simulink model "Encoder_Sim3"  (R2024b)
settings: Solver=FixedStepAuto  StartTime=0.0  StopTime=inf  FixedStep=0.01  RelTol=1e-3  EnableMultiTasking=on
libraries: stm32g4xxblockslib x4, stm32f4xxblockslib x3
settings Model: STM32="{\"EncoderBlockForG4\":[{\"ID\":\"Encoder_Sim3:80\"},{\"ID\":\"Encoder_Sim3:125\"},{\"ID\":\"Encoder_Sim3:137\"},{\"ID\":\"Encoder_Sim3:146\"}],\"DigitalPortRead\":[{\"ID\":\"Encoder_Sim3:75\"},{\"ID\":\"Encoder_Sim3:123\"},{\"ID\":\"Encoder_Sim3:135\"}]}"  SimulationMode=external  Creator=chant  LastModifiedBy=chant
settings OptimizationCC: DefaultParameterBehavior=Inlined  EnhancedBackFolding=on  PassReuseOutputArgsAs=Individual arguments  ZeroExternalMemoryAtStartup=off  ZeroInternalMemoryAtStartup=off  MaxStackSize=512  OptimizeBlockOrder=speed  DifferentSizesBufferReuse=on  OptimizationCustomize=off  EfficientTunableParamExpr=on
settings DebuggingCC: ParameterTunabilityLossMsg=error
settings HardwareCC: ProdBitPerPointer=32  ProdBitPerSizeT=32  ProdBitPerPtrDiffT=32  ProdLargestAtomicInteger=Long  ProdLargestAtomicFloat=Double  ProdWordSize=32  ProdLongLongMode=on  ProdHWDeviceType=ARM Compatible->ARM Cortex-M
settings SFSimCC: MATLABDynamicMemAlloc=off
settings RTWCC: Description=Embedded Coder  SystemTargetFile=ert.tlc  HardwareBoard=STM32G4xx Based  TemplateMakefile=ert_default_tmf  Toolchain=GNU Tools for ARM Embedded Processors
settings CodeAppCC: ForceParamTrailComments=on  IgnoreCustomStorageClasses=off  OperatorAnnotations=on  SimulinkDataObjDesc=on  SFDataObjDesc=on  InsertBlockDesc=on
settings ERTTargetCC: TargetLangStandard=C99 (ISO)  CodeReplacementLibrary=ARM Cortex-M  ExtModeTransport=3  ExtModeStaticAlloc=on  ExtModeStaticAllocSize=2048  ExtModeMexFile=ext_xcp  ExtModeIntrfLevel=Level2 - Open

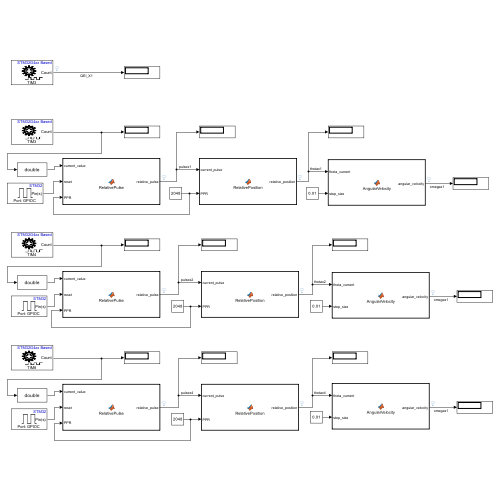
[thumbnail: Simulink's stored preview of the top-level diagram]
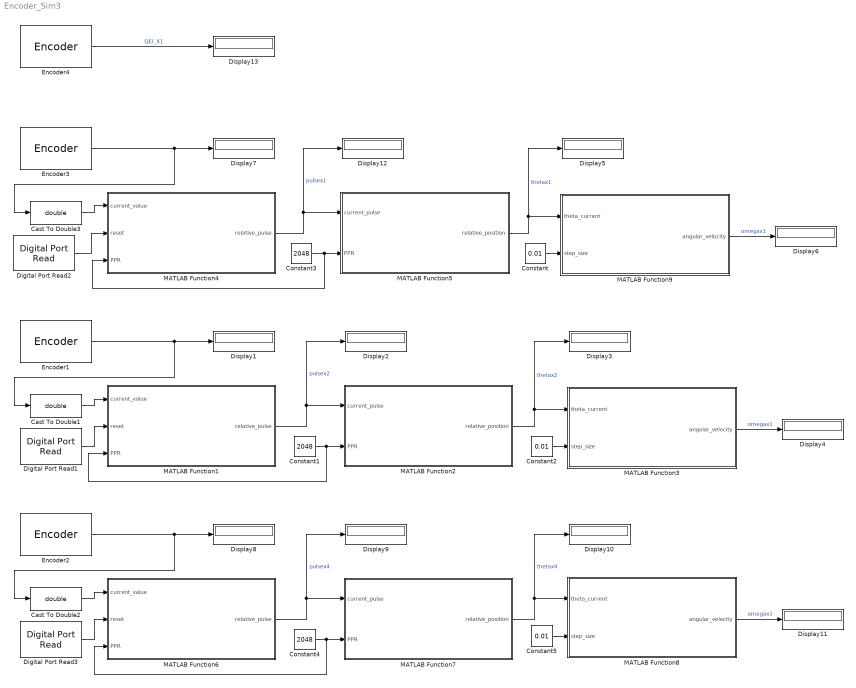
== system Encoder_Sim3 ==
  Cast To Double1 : DataTypeConversion  OutDataTypeStr=double  SaturateOnIntegerOverflow=off  RndMeth=Floor
  Cast To Double2 : DataTypeConversion  OutDataTypeStr=double  SaturateOnIntegerOverflow=off  RndMeth=Floor
  Cast To Double3 : DataTypeConversion  OutDataTypeStr=double  SaturateOnIntegerOverflow=off  RndMeth=Floor
  Constant : Constant  Value=0.01
  Constant1 : Constant  Value=2048
  Constant2 : Constant  Value=0.01
  Constant3 : Constant  Value=2048
  Constant4 : Constant  Value=2048
  Constant5 : Constant  Value=0.01
  Digital Port Read1 : stm32f4xxblockslib/Digital Port Read  PortName=GPIOC  PinNumber=[13]  ReadOperation=on  IOAsArray=on  SampleTime=-1  EnableSimPort=off  hoistedMaskSrc=ECSoC/ECSimCodegen/Digital Port Read
      settings: LibrarySourceBlock=stm32g4xxblockslib/Digital Port Read
  Digital Port Read2 : stm32f4xxblockslib/Digital Port Read  PortName=GPIOC  PinNumber=[13]  ReadOperation=on  IOAsArray=on  SampleTime=-1  EnableSimPort=off  hoistedMaskSrc=ECSoC/ECSimCodegen/Digital Port Read
      settings: LibrarySourceBlock=stm32g4xxblockslib/Digital Port Read
  Digital Port Read3 : stm32f4xxblockslib/Digital Port Read  PortName=GPIOC  PinNumber=[13]  ReadOperation=on  IOAsArray=on  SampleTime=-1  EnableSimPort=off  hoistedMaskSrc=ECSoC/ECSimCodegen/Digital Port Read
      settings: LibrarySourceBlock=stm32g4xxblockslib/Digital Port Read
  Display{1..13} (13 alike) : Display
  Encoder1 : stm32g4xxblockslib/Encoder  TimerModule=TIM4  EnableResetInput=off  OutputCountAfterFirstIndex=off  OutputValidIndex=off  OutputDirection=off  OutputStatus=off  SampleTime=-1
  Encoder2 : stm32g4xxblockslib/Encoder  TimerModule=TIM8  EnableResetInput=off  OutputCountAfterFirstIndex=off  OutputValidIndex=off  OutputDirection=off  OutputStatus=off  SampleTime=-1
  Encoder3 : stm32g4xxblockslib/Encoder  TimerModule=TIM3  EnableResetInput=off  OutputCountAfterFirstIndex=off  OutputValidIndex=off  OutputDirection=off  OutputStatus=off  SampleTime=-1
  Encoder4 : stm32g4xxblockslib/Encoder  TimerModule=TIM3  EnableResetInput=off  OutputCountAfterFirstIndex=off  OutputValidIndex=off  OutputDirection=off  OutputStatus=off  SampleTime=-1
  MATLAB Function1 : MATLAB Function  TreatAsAtomicUnit=on
  MATLAB Function2 : MATLAB Function  TreatAsAtomicUnit=on
  MATLAB Function3 : MATLAB Function  TreatAsAtomicUnit=on
  MATLAB Function4 : MATLAB Function  TreatAsAtomicUnit=on
  MATLAB Function5 : MATLAB Function  TreatAsAtomicUnit=on
  MATLAB Function6 : MATLAB Function  TreatAsAtomicUnit=on
  MATLAB Function7 : MATLAB Function  TreatAsAtomicUnit=on
  MATLAB Function8 : MATLAB Function  TreatAsAtomicUnit=on
  MATLAB Function9 : MATLAB Function  TreatAsAtomicUnit=on
  wires:
  Cast To Double3/1 -> MATLAB Function4/1(current_value)
  MATLAB Function9/1(angular_velocity) -> Display6/1  "omegax1"
  MATLAB Function5/1(relative_position) -> Display5/1, MATLAB Function9/1(theta_current)  "thetax1"
  Digital Port Read2/1 -> MATLAB Function4/2(reset)
  Encoder3/1 -> Display7/1, Cast To Double3/1
  Constant3/1 -> MATLAB Function4/3(PPR), MATLAB Function5/2(PPR)
  MATLAB Function4/1(relative_pulse) -> MATLAB Function5/1(current_pulse), Display12/1  "pulsex1"
  Constant/1 -> MATLAB Function9/2(step_size)
  Encoder1/1 -> Cast To Double1/1, Display1/1
  Digital Port Read1/1 -> MATLAB Function1/2(reset)
  Cast To Double1/1 -> MATLAB Function1/1(current_value)
  MATLAB Function1/1(relative_pulse) -> Display2/1, MATLAB Function2/1(current_pulse)  "pulsex2"
  Constant1/1 -> MATLAB Function1/3(PPR), MATLAB Function2/2(PPR)
  Constant2/1 -> MATLAB Function3/2(step_size)
  MATLAB Function2/1(relative_position) -> MATLAB Function3/1(theta_current), Display3/1  "thetax2"
  MATLAB Function3/1(angular_velocity) -> Display4/1  "omegax1"
  Cast To Double2/1 -> MATLAB Function6/1(current_value)
  Digital Port Read3/1 -> MATLAB Function6/2(reset)
  Encoder2/1 -> Display8/1, Cast To Double2/1
  Constant4/1 -> MATLAB Function6/3(PPR), MATLAB Function7/2(PPR)
  MATLAB Function6/1(relative_pulse) -> MATLAB Function7/1(current_pulse), Display9/1  "pulsex4"
  MATLAB Function8/1(angular_velocity) -> Display11/1  "omegax1"
  MATLAB Function7/1(relative_position) -> Display10/1, MATLAB Function8/1(theta_current)  "thetax4"
  Constant5/1 -> MATLAB Function8/2(step_size)
  Encoder4/1 -> Display13/1  "QEI_X1"

== matlab function Encoder_Sim3/MATLAB Function1 ==
  data: current_value input; relative_pulse output; reset input; PPR input
function relative_pulse = RelativePulse(current_value, reset, PPR)
    % Persistent variables to retain values across function calls
    persistent prev_value rollover_count max_value reset_flag pulse_offset

    % Initialize persistent variables on the first function call
    if isempty(prev_value)
        prev_value = 0;
    end
    if isempty(rollover_count)
        rollover_count = 0;
    end
    if isempty(max_value)
        max_value = 65535-(mod(65535, PPR)); % Set a default max value if not provided
    end
    if isempty(reset_flag)
        reset_flag = 0; % Track if reset has been triggered
    end
    if isempty(pulse_offset)
        pulse_offset = 0; % Offset to correct pulse on reset
    end

    % Set a default value for relative_pulse to avoid "undefined" errors
    relative_pulse = 0;

    % Threshold to detect overflow/underflow
    threshold = max_value / 2;

    % Detect overflow (encoder wrapped from high to low)
    if current_value < prev_value && (prev_value - current_value) > threshold
        rollover_count = rollover_count + 1;

    % Detect underflow (encoder wrapped from low to high)
    elseif current_value > prev_value && (current_value - prev_value) > threshold
        rollover_count = rollover_count - 1;
    end

    % Calculate true count (absolute pulse count)
    true_count = rollover_count * (max_value + 1) + current_value;

    % Homing logic: align to zero on reset
    if reset == 1 && reset_flag == 0
        % Set pulse_offset to the current true_count, so relative_pulse resets to 0
        pulse_offset = true_count;
        reset_flag = 1;  % Set the reset flag to avoid multiple resets
    elseif reset == 0
        % Clear the reset flag once the button is released
        reset_flag = 0;
    end

    % Calculate relative pulse with offset compensation
    relative_pulse = true_count - pulse_offset;

    % Update previous value for the next call
    prev_value = current_value;
end

== matlab function Encoder_Sim3/MATLAB Function2 ==
  data: current_pulse input; relative_position output; PPR input
function relative_position = RelativePosition(current_pulse, PPR)
    % Persistent variables to retain values across function calls
    persistent prev_pulse rollover_count max_value

    % Initialize persistent variables on the first function call
    if isempty(prev_pulse)
        prev_pulse = 0;
    end
    if isempty(rollover_count)
        rollover_count = 0;
    end
    if isempty(max_value)
        max_value = 23; % Maximum value for a 16-bit encoder
    end

    % Detect overflow (encoder wrapped from max to 0)
    if current_pulse < prev_pulse && (prev_pulse - current_pulse) > (max_value / 2)
        rollover_count = rollover_count + 1;

    % Detect underflow (encoder wrapped from 0 to max)
    elseif current_pulse > prev_pulse && (current_pulse - prev_pulse) > (max_value / 2)
        rollover_count = rollover_count - 1;
    end

    % Calculate true count (relative pulse)
    true_count = rollover_count * (max_value + 1) + current_pulse;

    % Calculate the relative position in radians (unlimited)
    relative_position = true_count * (2 * pi / PPR); % Convert to radians

    % Update previous value for the next call
    prev_pulse = current_pulse;
end

== matlab function Encoder_Sim3/MATLAB Function3 ==
  data: theta_current input; angular_velocity output; step_size input
function angular_velocity = AngularVelocity(theta_current, step_size)
    % Calculate angular velocity based on the fixed step size
    % Inputs:
    %   theta_current: The current angular position (in degrees)
    %   step_size: The fixed time step size (in seconds)

    % Persistent variable to store the previous position
    persistent theta_previous;

    % Initialize on the first call
    if isempty(theta_previous)
        theta_previous = theta_current;
        angular_velocity = 0;  % Start with zero angular velocity
        return;  % Exit on the first call
    end

    % Calculate the change in position (delta_theta)
    delta_theta = theta_current - theta_previous;

    % Calculate angular velocity (degrees per second)
    angular_velocity = delta_theta / step_size;

    % Update the previous position for the next call
    theta_previous = theta_current;
end

== matlab function Encoder_Sim3/MATLAB Function4 ==
  data: current_value input; relative_pulse output; reset input; PPR input
function relative_pulse = RelativePulse(current_value, reset, PPR)
    % Persistent variables to retain values across function calls
    persistent prev_value rollover_count max_value reset_flag pulse_offset

    % Initialize persistent variables on the first function call
    if isempty(prev_value)
        prev_value = 0;
    end
    if isempty(rollover_count)
        rollover_count = 0;
    end
    if isempty(max_value)
        max_value = 65535-(mod(65535, PPR)); % Set a default max value if not provided
    end
    if isempty(reset_flag)
        reset_flag = 0; % Track if reset has been triggered
    end
    if isempty(pulse_offset)
        pulse_offset = 0; % Offset to correct pulse on reset
    end

    % Set a default value for relative_pulse to avoid "undefined" errors
    relative_pulse = 0;

    % Threshold to detect overflow/underflow
    threshold = max_value / 2;

    % Detect overflow (encoder wrapped from high to low)
    if current_value < prev_value && (prev_value - current_value) > threshold
        rollover_count = rollover_count + 1;

    % Detect underflow (encoder wrapped from low to high)
    elseif current_value > prev_value && (current_value - prev_value) > threshold
        rollover_count = rollover_count - 1;
    end

    % Calculate true count (absolute pulse count)
    true_count = rollover_count * (max_value + 1) + current_value;

    % Homing logic: align to zero on reset
    if reset == 1 && reset_flag == 0
        % Set pulse_offset to the current true_count, so relative_pulse resets to 0
        pulse_offset = true_count;
        reset_flag = 1;  % Set the reset flag to avoid multiple resets
    elseif reset == 0
        % Clear the reset flag once the button is released
        reset_flag = 0;
    end

    % Calculate relative pulse with offset compensation
    relative_pulse = true_count - pulse_offset;

    % Update previous value for the next call
    prev_value = current_value;
end

== matlab function Encoder_Sim3/MATLAB Function5 ==
  data: current_pulse input; relative_position output; PPR input
function relative_position = RelativePosition(current_pulse, PPR)
    % Persistent variables to retain values across function calls
    persistent prev_pulse rollover_count max_value

    % Initialize persistent variables on the first function call
    if isempty(prev_pulse)
        prev_pulse = 0;
    end
    if isempty(rollover_count)
        rollover_count = 0;
    end
    if isempty(max_value)
        max_value = 23; % Maximum value for a 16-bit encoder
    end

    % Detect overflow (encoder wrapped from max to 0)
    if current_pulse < prev_pulse && (prev_pulse - current_pulse) > (max_value / 2)
        rollover_count = rollover_count + 1;

    % Detect underflow (encoder wrapped from 0 to max)
    elseif current_pulse > prev_pulse && (current_pulse - prev_pulse) > (max_value / 2)
        rollover_count = rollover_count - 1;
    end

    % Calculate true count (relative pulse)
    true_count = rollover_count * (max_value + 1) + current_pulse;

    % Calculate the relative position in radians (unlimited)
    relative_position = true_count * (2 * pi / PPR); % Convert to radians

    % Update previous value for the next call
    prev_pulse = current_pulse;
end

== matlab function Encoder_Sim3/MATLAB Function9 ==
  data: theta_current input; angular_velocity output; step_size input
function angular_velocity = AngularVelocity(theta_current, step_size)
    % Calculate angular velocity based on the fixed step size
    % Inputs:
    %   theta_current: The current angular position (in degrees)
    %   step_size: The fixed time step size (in seconds)

    % Persistent variable to store the previous position
    persistent theta_previous;

    % Initialize on the first call
    if isempty(theta_previous)
        theta_previous = theta_current;
        angular_velocity = 0;  % Start with zero angular velocity
        return;  % Exit on the first call
    end

    % Calculate the change in position (delta_theta)
    delta_theta = theta_current - theta_previous;

    % Calculate angular velocity (degrees per second)
    angular_velocity = delta_theta / step_size;

    % Update the previous position for the next call
    theta_previous = theta_current;
end

== matlab function Encoder_Sim3/MATLAB Function6 ==
  data: current_value input; relative_pulse output; reset input; PPR input
function relative_pulse = RelativePulse(current_value, reset, PPR)
    % Persistent variables to retain values across function calls
    persistent prev_value rollover_count max_value reset_flag pulse_offset

    % Initialize persistent variables on the first function call
    if isempty(prev_value)
        prev_value = 0;
    end
    if isempty(rollover_count)
        rollover_count = 0;
    end
    if isempty(max_value)
        max_value = 65535-(mod(65535, PPR)); % Set a default max value if not provided
    end
    if isempty(reset_flag)
        reset_flag = 0; % Track if reset has been triggered
    end
    if isempty(pulse_offset)
        pulse_offset = 0; % Offset to correct pulse on reset
    end

    % Set a default value for relative_pulse to avoid "undefined" errors
    relative_pulse = 0;

    % Threshold to detect overflow/underflow
    threshold = max_value / 2;

    % Detect overflow (encoder wrapped from high to low)
    if current_value < prev_value && (prev_value - current_value) > threshold
        rollover_count = rollover_count + 1;

    % Detect underflow (encoder wrapped from low to high)
    elseif current_value > prev_value && (current_value - prev_value) > threshold
        rollover_count = rollover_count - 1;
    end

    % Calculate true count (absolute pulse count)
    true_count = rollover_count * (max_value + 1) + current_value;

    % Homing logic: align to zero on reset
    if reset == 1 && reset_flag == 0
        % Set pulse_offset to the current true_count, so relative_pulse resets to 0
        pulse_offset = true_count;
        reset_flag = 1;  % Set the reset flag to avoid multiple resets
    elseif reset == 0
        % Clear the reset flag once the button is released
        reset_flag = 0;
    end

    % Calculate relative pulse with offset compensation
    relative_pulse = true_count - pulse_offset;

    % Update previous value for the next call
    prev_value = current_value;
end

== matlab function Encoder_Sim3/MATLAB Function7 ==
  data: current_pulse input; relative_position output; PPR input
function relative_position = RelativePosition(current_pulse, PPR)
    % Persistent variables to retain values across function calls
    persistent prev_pulse rollover_count max_value

    % Initialize persistent variables on the first function call
    if isempty(prev_pulse)
        prev_pulse = 0;
    end
    if isempty(rollover_count)
        rollover_count = 0;
    end
    if isempty(max_value)
        max_value = 23; % Maximum value for a 16-bit encoder
    end

    % Detect overflow (encoder wrapped from max to 0)
    if current_pulse < prev_pulse && (prev_pulse - current_pulse) > (max_value / 2)
        rollover_count = rollover_count + 1;

    % Detect underflow (encoder wrapped from 0 to max)
    elseif current_pulse > prev_pulse && (current_pulse - prev_pulse) > (max_value / 2)
        rollover_count = rollover_count - 1;
    end

    % Calculate true count (relative pulse)
    true_count = rollover_count * (max_value + 1) + current_pulse;

    % Calculate the relative position in radians (unlimited)
    relative_position = true_count * (2 * pi / PPR); % Convert to radians

    % Update previous value for the next call
    prev_pulse = current_pulse;
end

== matlab function Encoder_Sim3/MATLAB Function8 ==
  data: theta_current input; angular_velocity output; step_size input
function angular_velocity = AngularVelocity(theta_current, step_size)
    % Calculate angular velocity based on the fixed step size
    % Inputs:
    %   theta_current: The current angular position (in degrees)
    %   step_size: The fixed time step size (in seconds)

    % Persistent variable to store the previous position
    persistent theta_previous;

    % Initialize on the first call
    if isempty(theta_previous)
        theta_previous = theta_current;
        angular_velocity = 0;  % Start with zero angular velocity
        return;  % Exit on the first call
    end

    % Calculate the change in position (delta_theta)
    delta_theta = theta_current - theta_previous;

    % Calculate angular velocity (degrees per second)
    angular_velocity = delta_theta / step_size;

    % Update the previous position for the next call
    theta_previous = theta_current;
end
